simulink model "BiorlWalkingBipedRobot copy"  (R2023b)
settings: Solver=ode23t  StartTime=0.0  StopTime=inf  RelTol=1e-2  EnableMultiTasking=on
undefined symbols (not defined in the file or in its folder): foot_z, height_plane, init_angs_R, init_height, joint_stiffness, lower_leg_length, max_torque, plane_x, plane_y, Tf, Ts, upper_leg_length, wx0, wy0, X, Y, Z
libraries: sm_lib x38, nesl_utility x25, walkingRobotUtils x4, simulink x2, rllib x1
(part 2 of 2)

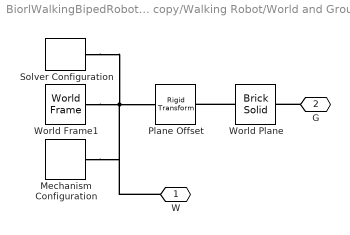
== system BiorlWalkingBipedRobot copy/Walking Robot/World and Ground ==
  Mechanism Configuration : sm_lib/Utilities/Mechanism Configuration  UniformGravity=Constant  GravityVector=[0 0 -9.80665]  GravityVectorUnits=m/s^2  LinearizationDelta=0.001  JointModeTransitionNonlinearIterations=2
  Plane Offset : sm_lib/Frames and Transforms/Rigid Transform  TranslationMethod=StandardAxis  TranslationStandardOffset=height_plane/2  TranslationStandardOffsetUnits=m  TranslationStandardAxis=-Z  TranslationCartesianOffset=[0 0 0]  TranslationCartesianOffsetUnits=m  TranslationROffset=0  TranslationROffsetUnits=m  TranslationZOffset=0  TranslationZOffsetUnits=m  TranslationThetaOffset=0  TranslationThetaOffsetUnits=deg  RotationMethod=None  RotationAngleUnits=deg  RotationStandardAxis=+Z  RotationAngle=0.0  RotationArbitraryAxis=[0 0 1]  FollAlignAxisA=+X  BaseAlignAxisA=+Y  FollAlignAxisB=+Y  BaseAlignAxisB=+Z  RotationSequenceAxes=FollowerAxes  RotationSequence=XYX  RotationSequenceAngles=[0 0 0]  RotationSequenceAnglesUnits=deg  RotationMatrix=[1 0 0; 0 1 0; 0 0 1]  Quaternion=[1 0 0 0]
  Solver Configuration : nesl_utility/Solver Configuration  PhysicalDomain=network_engine_domain  SubClassName=solver  LeftPortType=input  RightPortType=generic  Tones=[]  Harmonics=[]  SimulateNoise=off  Profile=off  UseLocalSampling=off  EnableSwitchedLinearOptims=on  FrequencyDomain=off  UseCCode=off  RelTol=0.001  AbsTol=1e-06  MinStep=1e-09  ToWorkspace=off  RevertToSquareIcSolve=off  NumHomotopyIterations=100  PhasorMode=off  PhasorModeNumHarmonics=1  ConsistencySolver=NEWTON_FTOL  IndexReductionMethod=DerivativeReplacement  DoDC=off  ResidualTolerance=1e-09  ConsistencyTolSource=GLOBAL  ConsistencyAbsTol=0.001  ConsistencyRelTol=0.001  ConsistencyTolFactor=0.001  UseLocalSolver=off  LocalSolverChoice=NE_TRAPEZOIDAL_ADVANCER  ResolveIndetEquations=on  FunctionEvalNumThread=1  LocalSolverSampleTime=Ts  DoFixedCost=off  MaxNonlinIter=3  MaxModeIter=2  ComputeImpulses=off  ImpulseIterations=2  LinearAlgebra=Sparse  LinearAlgebraNumThread=0  EquationFormulation=NE_TIME_EF  DelaysMemoryBudget=1024  AutomaticFiltering=on  FilteringTimeConstant=0.001  PartitionStorageMethod=AS_NEEDED  PartitionMemoryBudget=1024  PartitionMethod=FAST  MultibodyUseLocalSolver=off  MultibodyLocalSolverChoice=ODE1  MultibodyLocalSolverSampleTime=0.001
  World Frame1 : sm_lib/Frames and Transforms/World Frame
  World Plane : sm_lib/Body Elements/Brick Solid  GraphicAmbientColor=[0.15 0.15 0.15 1.0]  BasedOnType=Density  BrickDimensions="[plane_x plane_y  height_plane]"  BrickDimensionsUnits=m  CenterOfMass=[0 0 0]  CenterOfMassUnits=m  GraphicDiffuseColor=[1.0 1.0 0.8]  Density=density  DensityUnits=kg/(m^3)  DoExposeReferenceFrame=on  GraphicEmissiveColor=[0.0 0.0 0.0 1.0]  ExportEntireGeometry=on  SerializedFrames=<Frames/>  MarkerShape=Sphere  MarkerSize=10  GraphicType=FromGeometry  InertiaType=CalculateFromGeometry  Mass=1  MassUnits=kg  MomentsOfInertia=[1 1 1]  MomentsOfInertiaUnits=kg*m^2  GraphicOpacity=0.5  ProductsOfInertia=[0 0 0]  ProductsOfInertiaUnits=kg*m^2  GraphicShininess=75  GraphicSpecularColor=[0.5 0.5 0.5 1.0]  GraphicVisPropType=SimpleVisualProperties
  W : PMIOPort  Side=Left
  G : PMIOPort  Port=2  Side=Right
  connections:
  G/RConn1 -- World Plane/LConn1
  World Plane/RConn1 -- Plane Offset/RConn1
  Solver Configuration/RConn1 -- Plane Offset/LConn1 -- Mechanism Configuration/RConn1 -- W/RConn1 -- World Frame1/RConn1

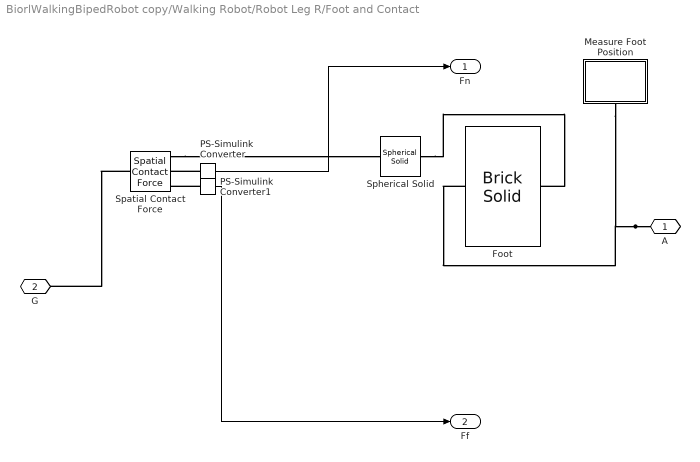
== system BiorlWalkingBipedRobot copy/Walking Robot/Robot Leg R/Foot and Contact ==
  Foot : sm_lib/Body Elements/Brick Solid  GraphicAmbientColor=[0.15 0.15 0.15 1.0]  BasedOnType=Density  BrickDimensions=[1 1 1]  BrickDimensionsUnits=cm  CenterOfMass=[0 0 0]  CenterOfMassUnits=m  GraphicDiffuseColor=[0.5 0.5 0.5]  Density=foot_density  DensityUnits=kg/(m^3)  DoExposeReferenceFrame=off  GraphicEmissiveColor=[0.0 0.0 0.0 1.0]  ExportEntireGeometry=off  SerializedFrames=<Frames><Frame><Id>Frame1</Id><Value><Name>F1</Name><Origin><Source>CenterOfMassFrame</Source><FeatureName></FeatureName></Origin><PrimaryAxis><DefinedDirection>+Z</DefinedDirection><Source>ReferenceFrame</Source><SourceDirection>+Z</SourceDirection><FeatureName></FeatureName></PrimaryAxis><SecondaryAxis><DefinedDirection>+X</DefinedDirection><Source>ReferenceFrame</Source><SourceDirection>+X</SourceDirection><FeatureName></FeatureName></SecondaryAxis></Value></Frame><Frame><Id>Frame5</Id><Value><Name>A</Name><Origin><Source>GeometricFeature</Source><FeatureName>+z surface</FeatureName></Origin><PrimaryAxis><DefinedDirection>+Z</DefinedDirection><Source>ReferenceFrame</Source><SourceDirection>-Y</SourceDirection><FeatureName></FeatureName></PrimaryAxis><SecondaryAxis><DefinedDirection>+X</DefinedDirection><Source>ReferenceFrame</Source><SourceDirection>+X</SourceDirection><FeatureName></FeatureName></SecondaryAxis></Value></Frame></Frames>  MarkerShape=Sphere  MarkerSize=10  GraphicType=FromGeometry  InertiaType=CalculateFromGeometry  Mass=1  MassUnits=kg  MomentsOfInertia=[1 1 1]  MomentsOfInertiaUnits=kg*m^2  GraphicOpacity=1.0  ProductsOfInertia=[0 0 0]  ProductsOfInertiaUnits=kg*m^2  GraphicShininess=75  GraphicSpecularColor=[0.5 0.5 0.5 1.0]  GraphicVisPropType=SimpleVisualProperties
  Measure Foot Position : Subsystem
  PS-Simulink Converter : nesl_utility/PS-Simulink Converter  PhysicalDomain=network_engine_domain  SubClassName=ps_output  LeftPortType=input  RightPortType=output  PseudoPeriodic=off  Frequencies=[]  VectorFormat=1-D array  Unit=inherit  AffineConversion=off
  PS-Simulink Converter1 : nesl_utility/PS-Simulink Converter  PhysicalDomain=network_engine_domain  SubClassName=ps_output  LeftPortType=input  RightPortType=output  PseudoPeriodic=off  Frequencies=[]  VectorFormat=1-D array  Unit=inherit  AffineConversion=off
  Spatial Contact Force : sm_lib/Forces and Torques/Spatial Contact Force  SenseContactBaseRotation=off  SenseContactBaseTranslation=off  CoefficientOfDynamicFriction=mu_k  CoefficientOfStaticFriction=mu_s  NormalDamping=contact_damping  NormalDampingUnits=N/(m/s)  SenseContactSignal=off  NormalStiffness=contact_stiffness  NormalStiffnessUnits=N/m  FrictionalCriticalVelocity=mu_vth  FrictionalCriticalVelocityUnits=m/s  ZeroCrossDetectContactStartAndEnd=off  SenseContactFollowerRotation=off  SenseContactFollowerTranslation=off  FrictionType=SmoothStickSlip  SenseFrictionalForceMagnitude=on  SenseNormalForceMagnitude=on  NormalForceType=SmoothSpringDamper  SenseNormalVelocity=off  SensePenetrationDepth=off  SenseSeparationDistance=off  SenseTangentialVelocity=off  NormalTransitionRegionWidth=1e-4  NormalTransitionRegionWidthUnits=m
  Spherical Solid : sm_lib/Body Elements/Spherical Solid  GraphicAmbientColor=[0.15 0.15 0.15 1.0]  BasedOnType=Mass  CenterOfMass=[0 0 0]  CenterOfMassUnits=m  GraphicDiffuseColor=[0.5 0.5 0.5]  Density=1000  DensityUnits=kg/m^3  DoExposeReferenceFrame=on  GraphicEmissiveColor=[0.0 0.0 0.0 1.0]  ExportEntireGeometry=on  SerializedExposedGeometries=<ExposedGeometries><ExposedGeometry><RawGeometryId>entire</RawGeometryId><ExposedGeometryId>G</ExposedGeometryId></ExposedGeometry></ExposedGeometries>  SerializedFrames=<Frames/>  MarkerShape=Sphere  MarkerSize=10  GraphicType=FromGeometry  InertiaType=CalculateFromGeometry  Mass=1  MassUnits=g  MomentsOfInertia=[1 1 1]  MomentsOfInertiaUnits=kg*m^2  GraphicOpacity=1.0  ProductsOfInertia=[0 0 0]  ProductsOfInertiaUnits=kg*m^2  GraphicShininess=75  GraphicSpecularColor=[0.5 0.5 0.5 1.0]  SphereRadius=foot_z/2  SphereRadiusUnits=cm  GraphicVisPropType=SimpleVisualProperties
  A : PMIOPort  Side=Right
  G : PMIOPort  Port=2  Side=Left
  Fn : Outport
  Ff : Outport  Port=2
  wires:
  PS-Simulink Converter/1 -> Fn/1
  PS-Simulink Converter1/1 -> Ff/1
  connections:
  Spatial Contact Force/LConn1 -- G/RConn1
  A/RConn1 -- Measure Foot Position/RConn1 -- Foot/RConn1
  PS-Simulink Converter/LConn1 -- Spatial Contact Force/RConn2
  PS-Simulink Converter1/LConn1 -- Spatial Contact Force/RConn3
  Spatial Contact Force/RConn1 -- Spherical Solid/LConn1
  Spherical Solid/RConn1 -- Foot/LConn1

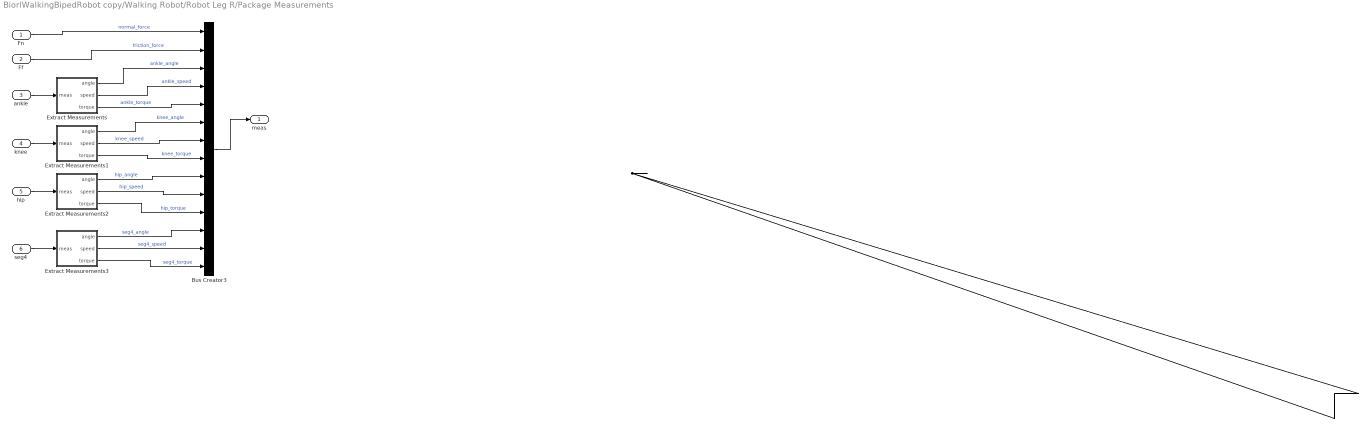
== system BiorlWalkingBipedRobot copy/Walking Robot/Robot Leg R/Package Measurements ==
  Fn : Inport
  Ff : Inport  Port=2
  ankle : Inport  Port=3
  knee : Inport  Port=4
  hip : Inport  Port=5
  seg4 : Inport  Port=6
  Bus Creator3 : BusCreator  Inputs=14
  Extract Measurements : Subsystem
  Extract Measurements1 : Subsystem
  Extract Measurements2 : Subsystem
  Extract Measurements3 : Subsystem
  meas : Outport  VectorParamsAs1DForOutWhenUnconnected=off
  wires:
  Fn/1 -> Bus Creator3/1  "normal_force"
  Ff/1 -> Bus Creator3/2  "friction_force"
  Extract Measurements2/3(torque) -> Bus Creator3/11  "hip_torque"
  Extract Measurements2/1(angle) -> Bus Creator3/9  "hip_angle"
  Extract Measurements1/3(torque) -> Bus Creator3/8  "knee_torque"
  Extract Measurements1/1(angle) -> Bus Creator3/6  "knee_angle"
  hip/1 -> Extract Measurements2/1(meas)
  knee/1 -> Extract Measurements1/1(meas)
  Extract Measurements/3(torque) -> Bus Creator3/5  "ankle_torque"
  Extract Measurements/1(angle) -> Bus Creator3/3  "ankle_angle"
  ankle/1 -> Extract Measurements/1(meas)
  Bus Creator3/1 -> meas/1
  Extract Measurements/2(speed) -> Bus Creator3/4  "ankle_speed"
  Extract Measurements1/2(speed) -> Bus Creator3/7  "knee_speed"
  Extract Measurements2/2(speed) -> Bus Creator3/10  "hip_speed"
  Extract Measurements3/1(angle) -> Bus Creator3/12  "seg4_angle"
  seg4/1 -> Extract Measurements3/1(meas)
  Extract Measurements3/2(speed) -> Bus Creator3/13  "seg4_speed"
  Extract Measurements3/3(torque) -> Bus Creator3/14  "seg4_torque"
  connections:
  ?

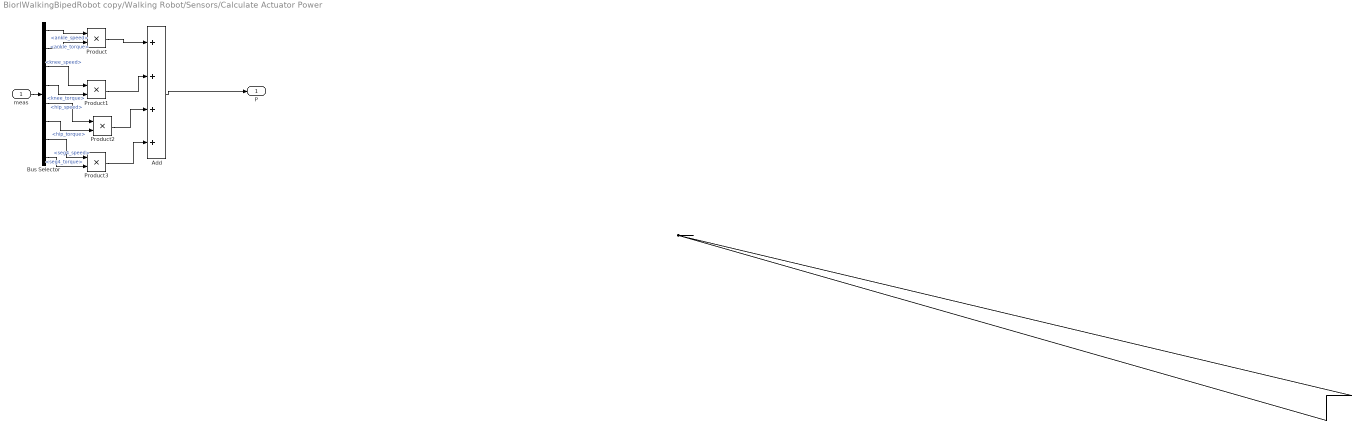
== system BiorlWalkingBipedRobot copy/Walking Robot/Sensors/Calculate Actuator Power ==
  meas : Inport
  Add : Sum  Inputs=4
  Bus Selector : BusSelector  OutputSignals=ankle_speed,ankle_torque,knee_speed,knee_torque,hip_speed,hip_torque,seg4_speed,seg4_torque
  Product{,1..3} (4 alike) : Product
  P : Outport  VectorParamsAs1DForOutWhenUnconnected=off
  wires:
  meas/1 -> Bus Selector/1
  Product2/1 -> Add/3
  Product1/1 -> Add/2
  Product/1 -> Add/1
  Add/1 -> P/1
  Bus Selector/1 -> Product/1  "<ankle_speed>"
  Bus Selector/2 -> Product/2  "<ankle_torque>"
  Bus Selector/3 -> Product1/1  "<knee_speed>"
  Bus Selector/4 -> Product1/2  "<knee_torque>"
  Bus Selector/5 -> Product2/1  "<hip_speed>"
  Bus Selector/6 -> Product2/2  "<hip_torque>"
  Bus Selector/7 -> Product3/1  "<seg4_speed>"
  Bus Selector/8 -> Product3/2  "<seg4_torque>"
  Product3/1 -> Add/4
  connections:
  ?

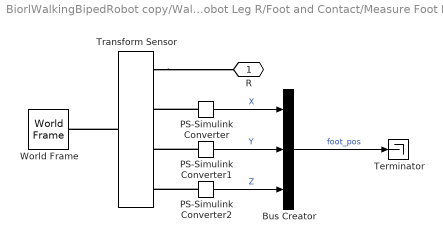
== system BiorlWalkingBipedRobot copy/Walking Robot/Robot Leg R/Foot and Contact/Measure Foot Position ==
  Bus Creator : BusCreator  Inputs=3
  PS-Simulink Converter : nesl_utility/PS-Simulink Converter  PhysicalDomain=network_engine_domain  SubClassName=ps_output  LeftPortType=input  RightPortType=output  PseudoPeriodic=off  Frequencies=[]  VectorFormat=1-D array  Unit=1  AffineConversion=off
  PS-Simulink Converter1 : nesl_utility/PS-Simulink Converter  PhysicalDomain=network_engine_domain  SubClassName=ps_output  LeftPortType=input  RightPortType=output  PseudoPeriodic=off  Frequencies=[]  VectorFormat=1-D array  Unit=1  AffineConversion=off
  PS-Simulink Converter2 : nesl_utility/PS-Simulink Converter  PhysicalDomain=network_engine_domain  SubClassName=ps_output  LeftPortType=input  RightPortType=output  PseudoPeriodic=off  Frequencies=[]  VectorFormat=1-D array  Unit=1  AffineConversion=off
  Terminator : Terminator
  Transform Sensor : sm_lib/Frames and Transforms/Transform Sensor  MeasurementFrame=World  RotationSequence=XYX  SenseAngle=off  SenseAxis=off  SenseQ=off  SenseR=off  SenseRotationSequence=off  SenseOmegaX=off  SenseOmegaY=off  SenseOmegaZ=off  SenseOmega=off  SenseQDot=off  SenseRDot=off  SenseRotationSequenceDot=off  SenseAlphaX=off  SenseAlphaY=off  SenseAlphaZ=off  SenseAlpha=off  SenseQDDot=off  SenseRDDot=off  SenseX=on  SenseY=on  SenseZ=on  SenseXYZ=off  SenseRad=off  SenseAzim=off  SenseDist=off  SenseInc=off  SenseXDot=off  SenseYDot=off  SenseZDot=off  SenseXYZDot=off  SenseRadDot=off  SenseAzimDot=off  SenseDistDot=off  SenseIncDot=off  SenseXDDot=off  SenseYDDot=off  SenseZDDot=off  SenseXYZDDot=off  SenseRadDDot=off  SenseAzimDDot=off  SenseDistDDot=off  SenseIncDDot=off
  World Frame : sm_lib/Frames and Transforms/World Frame
  R : PMIOPort  Side=Right
  wires:
  PS-Simulink Converter/1 -> Bus Creator/1  "X"
  PS-Simulink Converter1/1 -> Bus Creator/2  "Y"
  PS-Simulink Converter2/1 -> Bus Creator/3  "Z"
  Bus Creator/1 -> Terminator/1  "foot_pos"
  connections:
  Transform Sensor/LConn1 -- World Frame/RConn1
  Transform Sensor/RConn1 -- R/RConn1
  PS-Simulink Converter/LConn1 -- Transform Sensor/RConn2
  PS-Simulink Converter1/LConn1 -- Transform Sensor/RConn3
  PS-Simulink Converter2/LConn1 -- Transform Sensor/RConn4

== system BiorlWalkingBipedRobot copy/Walking Robot/Robot Leg R/Package Measurements/Extract Measurements ==
  meas : Inport
  Bus Selector : BusSelector  OutputSignals=angle,speed,torque
  angle : Outport  VectorParamsAs1DForOutWhenUnconnected=off
  speed : Outport  Port=2  VectorParamsAs1DForOutWhenUnconnected=off
  torque : Outport  Port=3  VectorParamsAs1DForOutWhenUnconnected=off
  wires:
  Bus Selector/1 -> angle/1  "<angle>"
  meas/1 -> Bus Selector/1
  Bus Selector/3 -> torque/1  "<torque>"
  Bus Selector/2 -> speed/1  "<speed>"

== system BiorlWalkingBipedRobot copy/Walking Robot/Robot Leg R/Package Measurements/Extract Measurements1 ==
  meas : Inport
  Bus Selector : BusSelector  OutputSignals=angle,speed,torque
  angle : Outport  VectorParamsAs1DForOutWhenUnconnected=off
  speed : Outport  Port=2  VectorParamsAs1DForOutWhenUnconnected=off
  torque : Outport  Port=3  VectorParamsAs1DForOutWhenUnconnected=off
  wires:
  Bus Selector/2 -> speed/1  "<speed>"
  Bus Selector/3 -> torque/1  "<torque>"
  meas/1 -> Bus Selector/1
  Bus Selector/1 -> angle/1  "<angle>"

== system BiorlWalkingBipedRobot copy/Walking Robot/Robot Leg R/Package Measurements/Extract Measurements2 ==
  meas : Inport
  Bus Selector : BusSelector  OutputSignals=angle,speed,torque
  angle : Outport  VectorParamsAs1DForOutWhenUnconnected=off
  speed : Outport  Port=2  VectorParamsAs1DForOutWhenUnconnected=off
  torque : Outport  Port=3  VectorParamsAs1DForOutWhenUnconnected=off
  wires:
  Bus Selector/1 -> angle/1  "<angle>"
  meas/1 -> Bus Selector/1
  Bus Selector/3 -> torque/1  "<torque>"
  Bus Selector/2 -> speed/1  "<speed>"

== system BiorlWalkingBipedRobot copy/Walking Robot/Robot Leg R/Package Measurements/Extract Measurements3 ==
  meas : Inport
  Bus Selector : BusSelector  OutputSignals=angle,speed,torque
  angle : Outport  VectorParamsAs1DForOutWhenUnconnected=off
  speed : Outport  Port=2  VectorParamsAs1DForOutWhenUnconnected=off
  torque : Outport  Port=3  VectorParamsAs1DForOutWhenUnconnected=off
  wires:
  Bus Selector/1 -> angle/1  "<angle>"
  meas/1 -> Bus Selector/1
  Bus Selector/3 -> torque/1  "<torque>"
  Bus Selector/2 -> speed/1  "<speed>"

== matlab function BiorlWalkingBipedRobot copy/Walking Robot/Sensors/Rotation Matrix to Yaw Pitch Roll ==
  data: q input; eul output
function eul = calcAttitude(q)

% Normalize the quaternions
q = bsxfun(@times, q, 1./sqrt(sum(q.^2,1)));
qw = q(1);
qx = q(2);
qy = q(3);
qz = q(4);

% Pre-allocate output
eul = zeros(3, 1, 'like', q);

aSinInput = -2*(qx.*qz-qw.*qy);
aSinInput(aSinInput > 1) = 1;
aSinInput(aSinInput < -1) = -1;

eul = [ atan2( 2*(qx.*qy+qw.*qz), qw.^2 + qx.^2 - qy.^2 - qz.^2 ); ...
    asin( aSinInput ); ...
    atan2( 2*(qy.*qz+qw.*qx), qw.^2 - qx.^2 - qy.^2 + qz.^2 )];
